simulink model "simulate"  (R2023a)
settings: Solver=VariableStepAuto  StartTime=0.0  StopTime=20.0  RelTol=1e-3
settings Model: Creator=zhs20  LastModifiedBy=zhs20

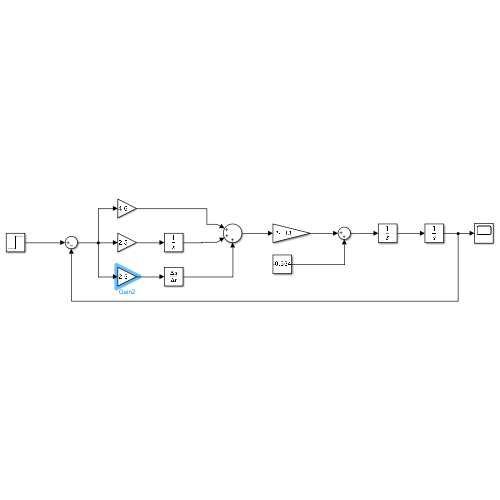
[thumbnail: Simulink's stored preview of the top-level diagram]
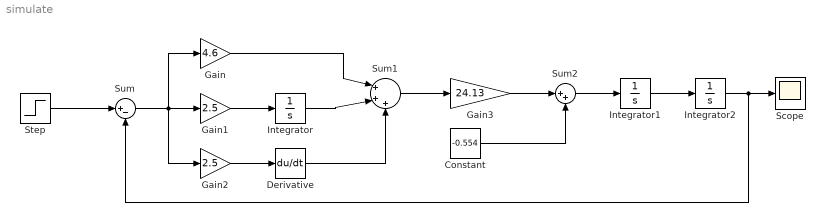
== system simulate ==
  Constant : Constant  Value=-0.554
  Derivative : Derivative
  Gain : Gain  Gain=4.6
  Gain1 : Gain  Gain=2.5
  Gain2 : Gain  Gain=2.5
  Gain3 : Gain  Gain=24.13
  Integrator : Integrator
  Integrator1 : Integrator
  Integrator2 : Integrator
  Scope : Scope
  Step : Step  After=0.3  SampleTime=0
  Sum : Sum  Inputs=|+-
  Sum1 : Sum  Inputs=|+++
  Sum2 : Sum  Inputs=|++
  wires:
  Sum2/1 -> Integrator1/1
  Gain2/1 -> Derivative/1
  Gain/1 -> Sum1/1
  Gain3/1 -> Sum2/1
  Integrator2/1 -> Sum/2, Scope/1
  Integrator1/1 -> Integrator2/1
  Constant/1 -> Sum2/2
  Sum1/1 -> Gain3/1
  Sum/1 -> Gain2/1, Gain1/1, Gain/1
  Step/1 -> Sum/1
  Integrator/1 -> Sum1/2
  Gain1/1 -> Integrator/1
  Derivative/1 -> Sum1/3
